simulink model "North_Country_Grid"  (R2025a)
settings: Solver=VariableStepAuto  StartTime=0.0  StopTime=10  RelTol=1e-3
PreLoadFcn:
  | Ts=50e-6;
InitFcn:
  | xInitial = WindFarmType4AverageModelInit;
  | Ts=50e-6;
undefined symbols (not defined in the file): D1, D11, Delta, DiscIntNeverNeededParam, find_system, Fnom_I, Fnom_R, Idc_nom, lagging, level, pulse, test_alpha, Vdc_nom, VLL_nom_I, VLL_nom_R
libraries: spsSecondOrderFilterLib x47, powerlib_extras x38, simulink x34, spsThreePhaseVIMeasurementLib x30, spsFirstOrderFilterLib x29, simulink_extras x26, spsabctodq0Lib x25, spsThreePhaseTransformerTwoWindingsLib x19, spsThreePhaseBreakerLib x18, spsThreePhasePISectionLineLib x17, spsControlledVoltageSourceLib x15, spsOnDelayLib x12
(part 8 of 18)

== system North_Country_Grid/Chateauguay HVDC Back-to-Back Converter/Inverter Control and Protection/Inverter Pole Control (Current//Voltage//Gamma)/Voltage Error ==
  note: Voltage Error
  Vd_ref : Inport
  Vd_meas : Inport  Port=2
  Block : Inport  Port=3
  Id_err : Inport  Port=4
  Enable (Held) : EnablePort  PropagateVarSize=During execution
  Constant1 : Constant  Value=0
  Constant2 : Constant  Value=0
  Constant3 : Constant  Value=Vd_marg
  Constant4 : Constant  Value=Id_marg
  First-Order Filter (T = 0.1) : spsFirstOrderFilterLib/First-Order Filter  FilterType=Lowpass  Tc=0.01  Ts=Ts  Initialize=on  Vac_Init=[0, 0, 60]  Vdc_Init=0  PlotResponse=off  FreqRange="[0,  200,  1]"
  MIN:eps MAX:inf : Saturate  UpperLimit=inf  LowerLimit=eps
  Math Function : Math  Operator=reciprocal  SignedPower=on
  Product1 : Product  Inputs=3  InputSameDT=on  SaturateOnIntegerOverflow=on  OutDataTypeStr=Inherit: Same as first input
  Saturation Dynamic : simulink/Discontinuities/Saturation Dynamic  OutMin=[]  OutMax=[]  OutDataTypeStr=Inherit: Same as second input  OutDataType=fixdt(1, 16)  OutScaling=2^-10  DoSatur=off
  Sum3 : Sum  Inputs=+--  InputSameDT=on  SaturateOnIntegerOverflow=on  OutDataTypeStr=Inherit: Same as first input
  Switch2 : Switch  Criteria=u2 > Threshold
  ERR_V : Outport  VectorParamsAs1DForOutWhenUnconnected=off
  wires:
  Saturation Dynamic/1 -> Product1/3
  Constant3/1 -> Product1/1
  Id_err/1 -> Saturation Dynamic/2
  First-Order Filter (T = 0.1)/1 -> Sum3/3  "dV"
  Product1/1 -> First-Order Filter (T = 0.1)/1
  Constant4/1 -> MIN:eps MAX:inf/1, Saturation Dynamic/1
  MIN:eps MAX:inf/1 -> Math Function/1
  Math Function/1 -> Product1/2
  Constant2/1 -> Saturation Dynamic/3
  Switch2/1 -> ERR_V/1  "ERR"
  Block/1 -> Switch2/2
  Constant1/1 -> Switch2/1
  Vd_meas/1 -> Sum3/2
  Vd_ref/1 -> Sum3/1
  Sum3/1 -> Switch2/3

== system North_Country_Grid/Chateauguay HVDC Back-to-Back Converter/Inverter Control and Protection/Inverter Pole Control (Current//Voltage//Gamma)/Voltage Regulator ==
  note: Voltage Regulator
  Max_i : Inport
  Min_i : Inport  Port=2
  ERR : Inport  Port=3
  Max_pi : Inport  Port=4
  Min_pi : Inport  Port=5
  Alpha_lin : Inport  Port=6
  Max_lin : Inport  Port=7
  Min_lin : Inport  Port=8
  Inv : Inport  Port=9
  Enable (Held) : EnablePort  PropagateVarSize=During execution
  PI Regulator with external limits and linrarized Kp (Discrete) : Subsystem  mask(PI Regulator  With  External  Limits (Discrete)){Kp=Kp_V, Ki=Ki_V, IC_i=ICi_V, On_lin=on, pas=Ts}
      mask prompts: Kp "Kp (deg/pu):"; Ki "Ki (deg/pu/s):"; IC_i "Integrator Initial Condition (deg):"; On_lin "Linearization  (On)"; pas "Sample time (s):"
      mask help: For the linearization it is important to specifie the mode of operation i.e. rectifier or inverter (negation of rectifier).
      mask Display: disp('PI Regulator\nWith external limits\n(Linearized Kp)\n(Discrete)\n\n')
  Alpha_ord : Outport  VectorParamsAs1DForOutWhenUnconnected=off
  wires:
  Inv/1 -> PI Regulator with external limits and linrarized Kp (Discrete)/9(Inv)
  Min_lin/1 -> PI Regulator with external limits and linrarized Kp (Discrete)/8(Min_lin)
  Max_lin/1 -> PI Regulator with external limits and linrarized Kp (Discrete)/7(Max_lin)
  Alpha_lin/1 -> PI Regulator with external limits and linrarized Kp (Discrete)/6(Alpha_lin)
  Min_pi/1 -> PI Regulator with external limits and linrarized Kp (Discrete)/5(Min_pi)
  Max_pi/1 -> PI Regulator with external limits and linrarized Kp (Discrete)/4(Max_pi)
  ERR/1 -> PI Regulator with external limits and linrarized Kp (Discrete)/3(ERR)
  Min_i/1 -> PI Regulator with external limits and linrarized Kp (Discrete)/2(Min_i)
  Max_i/1 -> PI Regulator with external limits and linrarized Kp (Discrete)/1(Max_i)
  PI Regulator with external limits and linrarized Kp (Discrete)/1(Alpha_ord) -> Alpha_ord/1

== system North_Country_Grid/Chateauguay HVDC Back-to-Back Converter/Inverter Control and Protection/Inverter Pole Control (Current//Voltage//Gamma)/Voltage dependent Current Order Limiter ==
  note: Voltage dependent Current Order Limiter (VDCOL) (Discrete)
  Id_ref (pu) : Inport
  Vd (pu) : Inport  Port=2
  Constant : Constant  Value=Id_min
  Constant1 : Constant  Value=Vd_min
  Constant2 : Constant  Value=Vd_seuil
  Constant3 : Constant
  Constant4 : Constant
  Constant5 : Constant  Value=Tu
  Logical Operator : Logic  Operator=NOT
  Low Pass (IC = 1.0) : Subsystem  mask(Low Pass Filter With Reset (discrete: Zoh method, Forward Euler)){ic=1, dt=Ts}
      mask prompts: ic "Initial condition:"; dt "Sample time (s)"
      mask help:
      | The output will be reset to the input value (Time constant = 0)  during the input (2) is True. The Time constant (T) is defined by
      | input (3).
      mask Display:
      | plot(0,0,100,100,[90,80,70,60,50,40,29,20,10],[60,55,52,55,60,65,67,65,60],[89,80,71,60,50,40,30,20,10],[40,35,32,35,40,45,47,45,40],[56,44],[70,50]);
      | disp('\n\nD')
  Math Function : Math  Operator=reciprocal  SignedPower=on
  Max = 10 Min=Id_min_abs : Saturate  UpperLimit=10  LowerLimit=Id_min_abs
  MinMax2 : MinMax  Function=max  Inputs=2  InputSameDT=on  SaturateOnIntegerOverflow=on
  MinMax3 : MinMax  Inputs=2  InputSameDT=on  SaturateOnIntegerOverflow=on
  Product{,1..4} (5 alike) : Product  InputSameDT=on  SaturateOnIntegerOverflow=on  OutDataTypeStr=Inherit: Same as first input
  Relational Operator : RelationalOperator
  Sum : Sum  Inputs=+-  InputSameDT=on  SaturateOnIntegerOverflow=on  OutDataTypeStr=Inherit: Same as first input
  Sum1 : Sum  Inputs=+-  InputSameDT=on  SaturateOnIntegerOverflow=on  OutDataTypeStr=Inherit: Same as first input
  Sum2 : Sum  Inputs=+-  InputSameDT=on  SaturateOnIntegerOverflow=on  OutDataTypeStr=Inherit: Same as first input
  Sum3 : Sum  InputSameDT=on  SaturateOnIntegerOverflow=on  OutDataTypeStr=Inherit: Same as first input
  Unit Delay : UnitDelay  SampleTime=Ts  HasFrameUpgradeWarning=on
  Id_ref_lim : Outport  InitialOutput=0  VectorParamsAs1DForOutWhenUnconnected=off
  Vd_filt : Outport  Port=2  InitialOutput=0  VectorParamsAs1DForOutWhenUnconnected=off
  wires:
  Relational Operator/1 -> Unit Delay/1
  Max = 10 Min=Id_min_abs/1 -> MinMax2/2
  MinMax2/1 -> MinMax3/2
  Product1/1 -> MinMax2/1  "Idref_lim"
  Constant2/1 -> Product3/1, Sum1/1
  Product/1 -> Product3/2, Product2/1  "A"
  Product3/1 -> Sum2/2
  MinMax3/1 -> Id_ref_lim/1
  Id_ref (pu)/1 -> Product4/2, MinMax3/1, Product1/1
  Product4/1 -> Max = 10 Min=Id_min_abs/1  "min"
  Constant/1 -> Product4/1, Sum/2
  Sum3/1 -> Product1/2
  Product2/1 -> Sum3/2
  Sum2/1 -> Sum3/1  "B"
  Constant4/1 -> Sum2/1
  Math Function/1 -> Product/2
  Sum/1 -> Product/1
  Sum1/1 -> Math Function/1
  Constant1/1 -> Sum1/2
  Constant3/1 -> Sum/1
  Constant5/1 -> Low Pass (IC = 1.0)/3(T)
  Low Pass (IC = 1.0)/1(Out) -> Vd_filt/1, Relational Operator/2, Product2/2
  Vd (pu)/1 -> Relational Operator/1, Low Pass (IC = 1.0)/1(In)
  Unit Delay/1 -> Logical Operator/1
  Logical Operator/1 -> Low Pass (IC = 1.0)/2(R)

== system North_Country_Grid/Chateauguay HVDC Back-to-Back Converter/Inverter Control and Protection/Inverter Pole Control (Current//Voltage//Gamma)/alpha_init ==
  In1 : Inport  PortDimensions=1
  IC : InitialCondition  Value=min([ICi_V,ICi_I,ICi_G])
  Out1 : Outport  VectorParamsAs1DForOutWhenUnconnected=off
  wires:
  IC/1 -> Out1/1
  In1/1 -> IC/1

== system North_Country_Grid/Chateauguay HVDC Back-to-Back Converter/Inverter Control and Protection/Inverter Protections/Commutation Failure Prevention Control (CFPREV) ==
  note: Commutation failure Prevention Control Module (CFPREV)
  Uabc (pu) : Inport
  C : Constant  Value=STATE
  CFPREV : Subsystem  TreatAsAtomicUnit=on
  AMIN_CFPREV (deg) : Outport  VectorParamsAs1DForOutWhenUnconnected=off
  wires:
  C/1 -> CFPREV/Enable
  Uabc (pu)/1 -> CFPREV/1(Uabc (pu))
  CFPREV/1(AMIN_CFPREV (deg)) -> AMIN_CFPREV (deg)/1

== system North_Country_Grid/Chateauguay HVDC Back-to-Back Converter/Inverter Control and Protection/Inverter Protections/Informations ==
  note: The CFPREV  mitigates commutation failures due to AC voltage dips. After a fault detection (three-phase or
      | one-phase) an angle value (AMIN_CFPREV) is sent to the converter control in order to be deducted from the
      | maximum delay angle limit (alpha_max). In practice, the commutation margin is consequently enlarged
      | reducing therefore the risk of commutation failures (note 1).
  note: The Commutation failure prevention control (CFPREV) and the Low AC voltage detection (LACVD)
      | constitutes the protective functions at the rinverter.
  note: The LACVD detects a low AC voltage condition on the inverter commutation bus and sends a signal
      | (Lock) to the DCPROT (in the rectifier) in order to prevent the detection of a DC fault when the drop in
      | the DC voltage is due to a fault on the AC side. The LACVD at the irectifier sends also a signal to
      | lock the DCPROT for the same reason.
  note: DESCRIPTION
  note: DC Protections - Inverter
  note: NOTE 1: Result of a failure of the incoming valve to take over the direct current before the commutating voltage reverses its polarity.

== system North_Country_Grid/Chateauguay HVDC Back-to-Back Converter/Inverter Control and Protection/Inverter Protections/Low  AC Voltage Detection (LACVD) ==
  note: Low AC Voltage Detection
  Uac (pu) : Inport
  Enable (Held) : EnablePort  PropagateVarSize=During execution  ShowOutputPort=on
  C : Constant  Value=STATE
  LACVD : Subsystem  TreatAsAtomicUnit=on
  Logical Operator : Logic  AllPortsSameDT=off
  Low_AC_Voltage : Outport  VectorParamsAs1DForOutWhenUnconnected=off
  wires:
  Uac (pu)/1 -> LACVD/1(Uac (pu))
  LACVD/1(Low_AC_Voltage) -> Low_AC_Voltage/1
  Enable (Held)/1 -> Logical Operator/1
  Logical Operator/1 -> LACVD/Enable
  C/1 -> Logical Operator/2

== system North_Country_Grid/Chateauguay HVDC Back-to-Back Converter/Inverter Control and Protection/Inverter Protections/Udio_6p ==
  note: Three-phase full-wave rectification
  Uabc (pu) : Inport
  MinMax : MinMax  Function=max  InputSameDT=on  SaturateOnIntegerOverflow=on
  MinMax1 : MinMax  InputSameDT=on  SaturateOnIntegerOverflow=on
  Sum : Sum  Inputs=+-  InputSameDT=on  SaturateOnIntegerOverflow=on  OutDataTypeStr=Inherit: Same as first input
  conversion pu ac->dc : Gain  Gain=pi/(3*sqrt(3))  SaturateOnIntegerOverflow=on  OutDataTypeStr=Inherit: Same as input  ParamDataTypeStr=Inherit: Same as input
  Udio_6p : Outport  VectorParamsAs1DForOutWhenUnconnected=off
  wires:
  conversion pu ac->dc/1 -> Udio_6p/1
  Sum/1 -> conversion pu ac->dc/1
  Uabc (pu)/1 -> MinMax1/1, MinMax/1
  MinMax/1 -> Sum/1
  MinMax1/1 -> Sum/2

== system North_Country_Grid/Chateauguay HVDC Back-to-Back Converter/Master Control/Start//Stop/S1 ==
  Start : Inport
  Down : Constant  Value=0
  Ramp : FromWorkspace  VariableName="[T_ramp,  U_ramp]"  SampleTime=Ts  ZeroCross=off
  Start-Stop Ramp : RateLimiter  RisingSlewLimit=SS_ramp  FallingSlewLimit=-SS_ramp
  Sum : Sum  InputSameDT=on  SaturateOnIntegerOverflow=on  OutDataTypeStr=Inherit: Same as first input
  Switch : Switch  Criteria=u2 > Threshold  InputSameDT=off
  UP : Constant  Value=Min_ref
  Out1 : Outport  InitialOutput=0  VectorParamsAs1DForOutWhenUnconnected=off
  wires:
  Sum/1 -> Out1/1
  Ramp/1 -> Sum/1
  Start/1 -> Switch/2
  Switch/1 -> Start-Stop Ramp/1
  Down/1 -> Switch/3
  UP/1 -> Switch/1
  Start-Stop Ramp/1 -> Sum/2

== system North_Country_Grid/Chateauguay HVDC Back-to-Back Converter/Rectifier Control and Protection/Rectifier Pole Control (Current)/Alpha Control ==
  note: Alpha Control
  Forced_alpha : Inport
  D_alpha : Inport  Port=2
  Constant1 : Constant  Value=alpha_min
  Constant2 : Constant  Value=alpha_max
  Constant3 : Constant  Value=test_alpha
  Data Type Conversion : DataTypeConversion  OutDataTypeStr=boolean
  Logical Operator : Logic  Operator=OR
  "Rate Limiter (Rate limit) " : RateLimiter  RisingSlewLimit=PRate_fix  FallingSlewLimit=NRate_fix
  "Rate Limiter (Rate limit)    " : RateLimiter  RisingSlewLimit=PRate_fix  FallingSlewLimit=NRate_fix
  Sum : Sum  Inputs=-+  InputSameDT=on  SaturateOnIntegerOverflow=on  OutDataTypeStr=Inherit: Same as first input
  Switch : Switch  Criteria=u2 > Threshold
  Switch1 : Switch  Criteria=u2 > Threshold
  fixed alpha (deg) : Constant  Value=alpha_fix
  Max_i : Outport  VectorParamsAs1DForOutWhenUnconnected=off
  Min_i : Outport  Port=2  VectorParamsAs1DForOutWhenUnconnected=off
  wires:
  "Rate Limiter (Rate limit)    "/1 -> Min_i/1
  "Rate Limiter (Rate limit) "/1 -> Max_i/1
  D_alpha/1 -> Sum/1
  Sum/1 -> Switch/3
  Constant2/1 -> Sum/2
  Constant3/1 -> Logical Operator/1
  Logical Operator/1 -> Switch/2, Switch1/2
  Constant1/1 -> Switch1/3
  Switch/1 -> "Rate Limiter (Rate limit) "/1
  Switch1/1 -> "Rate Limiter (Rate limit)    "/1
  fixed alpha (deg)/1 -> Switch/1, Switch1/1
  Forced_alpha/1 -> Data Type Conversion/1
  Data Type Conversion/1 -> Logical Operator/2

== system North_Country_Grid/Chateauguay HVDC Back-to-Back Converter/Rectifier Control and Protection/Rectifier Pole Control (Current)/Control Mode  ==
  note: AMIN
  note: CONTROL MODE (#):
      |
      | 0) Blocked
      | 1) Current control
      | 2) Voltage control
      | 3) Alpha minimum limitation
      | 4) Alpha maximum limitation
      | 5) Forced or constant Alpha
      | 6) Gamma control
  "a_ord_i " : Inport
  a_ord_v : Inport  Port=2
  a_ord_g : Inport  Port=3
  alpha_ord : Inport  Port=4
  Max_i : Inport  Port=5
  Min_i : Inport  Port=6
  Block : Inport  Port=7
  C : Constant  Value=0
  Data Type Conversion{1..6} (6 alike) : DataTypeConversion  OutDataTypeStr=double  SaturateOnIntegerOverflow=off  RndMeth=Floor
  Gain1 : Gain  Gain=3  OutDataTypeStr=double  SaturateOnIntegerOverflow=on  ParamDataTypeStr=Inherit: Same as input
  Gain2 : Gain  Gain=4  OutDataTypeStr=double  SaturateOnIntegerOverflow=on  ParamDataTypeStr=Inherit: Same as input
  Gain3 : Gain  Gain=2  OutDataTypeStr=double  SaturateOnIntegerOverflow=on  ParamDataTypeStr=Inherit: Same as input
  Gain4 : Gain  Gain=5  OutDataTypeStr=double  SaturateOnIntegerOverflow=on  ParamDataTypeStr=Inherit: Same as input
  Gain5 : Gain  Gain=6  OutDataTypeStr=double  SaturateOnIntegerOverflow=on  ParamDataTypeStr=Inherit: Same as input
  Logical Operator{,1,3,10} (4 alike) : Logic
  Logical Operator2 : Logic  Inputs=3
  Logical Operator4 : Logic  Operator=OR
  Logical Operator{5..7,9} (4 alike) : Logic  Operator=NOT
  Logical Operator8 : Logic  Operator=OR
  MinMax : MinMax  Inputs=2  InputSameDT=on  SaturateOnIntegerOverflow=on
  MinMax1 : MinMax  Inputs=2  InputSameDT=on  SaturateOnIntegerOverflow=on
  Relational Operator : RelationalOperator  Operator=<=
  Relational Operator1 : RelationalOperator  Operator=<=
  Relational Operator2 : RelationalOperator
  Relational Operator3 : RelationalOperator  Operator=<
  Relational Operator4 : RelationalOperator  Operator===
  Sum : Sum  Inputs=++++++  InputSameDT=on  SaturateOnIntegerOverflow=on  OutDataTypeStr=Inherit: Same as first input
  Switch : Switch  Criteria=u2 > Threshold
  mode : Outport  VectorParamsAs1DForOutWhenUnconnected=off
  wires:
  Data Type Conversion6/1 -> Gain4/1
  Data Type Conversion5/1 -> Gain2/1
  Data Type Conversion4/1 -> Gain1/1
  Data Type Conversion3/1 -> Gain5/1
  Data Type Conversion2/1 -> Gain3/1
  Data Type Conversion1/1 -> Sum/1
  Switch/1 -> mode/1
  Logical Operator5/1 -> Logical Operator3/2, Logical Operator/2, Logical Operator10/2
  Logical Operator7/1 -> Logical Operator2/3, Logical Operator1/2
  Gain4/1 -> Sum/5
  Logical Operator1/1 -> Data Type Conversion4/1
  Relational Operator4/1 -> Logical Operator7/1, Data Type Conversion6/1  "AFOR"
  Max_i/1 -> Relational Operator4/2, Relational Operator2/2
  Min_i/1 -> Relational Operator4/1, Relational Operator1/2
  Gain2/1 -> Sum/4
  Gain1/1 -> Sum/3
  Logical Operator2/1 -> Data Type Conversion5/1
  Logical Operator6/1 -> Logical Operator2/1
  Relational Operator2/1 -> Logical Operator2/2, Logical Operator4/2  "AMAX"
  Logical Operator4/1 -> Logical Operator5/1
  Relational Operator1/1 -> Logical Operator1/1, Logical Operator6/1, Logical Operator4/1
  alpha_ord/1 -> Relational Operator2/1, Relational Operator1/1  "alpha_ord"
  Logical Operator/1 -> Data Type Conversion2/1
  Relational Operator3/1 -> Logical Operator/1, Logical Operator8/2  "AVR"
  Gain3/1 -> Sum/2
  Logical Operator3/1 -> Data Type Conversion1/1
  Relational Operator/1 -> Logical Operator3/1, Logical Operator8/1  "ACR"
  "a_ord_i "/1 -> Relational Operator/1, MinMax1/1
  Block/1 -> Switch/2
  Sum/1 -> Switch/3
  C/1 -> Switch/1
  a_ord_v/1 -> MinMax/1, Relational Operator3/1
  a_ord_g/1 -> MinMax/2, MinMax1/2
  MinMax/1 -> Relational Operator/2
  Logical Operator8/1 -> Logical Operator9/1
  Gain5/1 -> Sum/6
  MinMax1/1 -> Relational Operator3/2
  Logical Operator9/1 -> Logical Operator10/1  "AGR"
  Logical Operator10/1 -> Data Type Conversion3/1

== system North_Country_Grid/Chateauguay HVDC Back-to-Back Converter/Rectifier Control and Protection/Rectifier Pole Control (Current)/Current Regulator ==
  note: Current Regulator
  Max_i : Inport
  Min_i : Inport  Port=2
  ERR : Inport  Port=3
  Max_pi : Inport  Port=4
  Min_pi : Inport  Port=5
  Alpha_lin : Inport  Port=6
  Max_lin : Inport  Port=7
  Min_lin : Inport  Port=8
  Inv : Inport  Port=9
  PI Regulator with external limits and linrarized Kp (Discrete) : Subsystem  mask(PI Regulator  With  External  Limits (Discrete)){Kp=Kp_I, Ki=Ki_I, IC_i=ICi_I, On_lin=on, pas=Ts}
      mask prompts: Kp "Kp (deg/pu):"; Ki "Ki (deg/pu/s):"; IC_i "Integrator Initial Condition (deg):"; On_lin "Linearization  (On)"; pas "Sample time (s):"
      mask help: For the linearization it is important to specifie the mode of operation i.e. rectifier or inverter (negation of rectifier).
      mask Display: disp('PI Regulator\nWith external limits\n(Linearized Kp)\n(Discrete)\n\n')
  Alpha_ord : Outport  VectorParamsAs1DForOutWhenUnconnected=off
  wires:
  PI Regulator with external limits and linrarized Kp (Discrete)/1(Alpha_ord) -> Alpha_ord/1
  Max_i/1 -> PI Regulator with external limits and linrarized Kp (Discrete)/1(Max_i)
  Min_i/1 -> PI Regulator with external limits and linrarized Kp (Discrete)/2(Min_i)
  ERR/1 -> PI Regulator with external limits and linrarized Kp (Discrete)/3(ERR)
  Max_pi/1 -> PI Regulator with external limits and linrarized Kp (Discrete)/4(Max_pi)
  Min_pi/1 -> PI Regulator with external limits and linrarized Kp (Discrete)/5(Min_pi)
  Alpha_lin/1 -> PI Regulator with external limits and linrarized Kp (Discrete)/6(Alpha_lin)
  Max_lin/1 -> PI Regulator with external limits and linrarized Kp (Discrete)/7(Max_lin)
  Min_lin/1 -> PI Regulator with external limits and linrarized Kp (Discrete)/8(Min_lin)
  Inv/1 -> PI Regulator with external limits and linrarized Kp (Discrete)/9(Inv)

== system North_Country_Grid/Chateauguay HVDC Back-to-Back Converter/Rectifier Control and Protection/Rectifier Pole Control (Current)/Gamma Error ==
  note: Gamma Error
  G_ref : Inport
  G_meas : Inport  Port=2
  Block : Inport  Port=3
  Id_err : Inport  Port=4
  Enable (Held) : EnablePort  PropagateVarSize=During execution
  Constant1 : Constant  Value=0
  Constant2 : Constant  Value=0
  Constant3 : Constant  Value=G_marg
  Constant4 : Constant  Value=Id_marg
  First-Order Filter (T=0.01) : spsFirstOrderFilterLib/First-Order Filter  FilterType=Lowpass  Tc=0.01  Ts=Ts  Initialize=off  Vac_Init=[0, 0, 60]  Vdc_Init=0  PlotResponse=off  FreqRange="[0,  200,  1]"
  MIN:eps MAX:inf : Saturate  UpperLimit=inf  LowerLimit=eps
  Math Function : Math  Operator=reciprocal  SignedPower=on
  Product1 : Product  Inputs=3  InputSameDT=on  SaturateOnIntegerOverflow=on  OutDataTypeStr=Inherit: Same as first input
  Saturation Dynamic : simulink/Discontinuities/Saturation Dynamic  OutMin=[]  OutMax=[]  OutDataTypeStr=Inherit: Same as second input  OutDataType=fixdt(1, 16)  OutScaling=2^-10  DoSatur=off
  Sum3 : Sum  Inputs=-+-  InputSameDT=on  SaturateOnIntegerOverflow=on  OutDataTypeStr=Inherit: Same as first input
  Switch2 : Switch  Criteria=u2 > Threshold
  ERR_G : Outport  VectorParamsAs1DForOutWhenUnconnected=off
  wires:
  Saturation Dynamic/1 -> Product1/3
  Sum3/1 -> Switch2/3
  G_ref/1 -> Sum3/1
  G_meas/1 -> Sum3/2
  Constant1/1 -> Switch2/1
  Block/1 -> Switch2/2
  Switch2/1 -> ERR_G/1  "ERR"
  Constant2/1 -> Saturation Dynamic/3
  Math Function/1 -> Product1/2
  MIN:eps MAX:inf/1 -> Math Function/1
  Constant4/1 -> MIN:eps MAX:inf/1, Saturation Dynamic/1
  Product1/1 -> First-Order Filter (T=0.01)/1
  First-Order Filter (T=0.01)/1 -> Sum3/3  "dG"
  Id_err/1 -> Saturation Dynamic/2
  Constant3/1 -> Product1/1

== system North_Country_Grid/Chateauguay HVDC Back-to-Back Converter/Rectifier Control and Protection/Rectifier Pole Control (Current)/Gamma Regulator ==
  note: Gamma Regulator
  Max_i : Inport
  Min_i : Inport  Port=2
  ERR : Inport  Port=3
  Max_pi : Inport  Port=4
  Min_pi : Inport  Port=5
  Alpha_lin : Inport  Port=6
  Max_lin : Inport  Port=7
  Min_lin : Inport  Port=8
  Inv : Inport  Port=9
  Enable (Held) : EnablePort  PropagateVarSize=During execution
  PI Regulator with external limits and linrarized Kp (Discrete)1 : Subsystem  mask(PI Regulator  With  External  Limits (Discrete)){Kp=Kp_G, Ki=Ki_G, IC_i=ICi_G, On_lin=on, pas=Ts}
      mask prompts: Kp "Kp (deg/pu):"; Ki "Ki (deg/pu/s):"; IC_i "Integrator Initial Condition (deg):"; On_lin "Linearization  (On)"; pas "Sample time (s):"
      mask help: For the linearization it is important to specifie the mode of operation i.e. rectifier or inverter (negation of rectifier).
      mask Display: disp('PI Regulator\nWith external limits\n(Linearized Kp)\n(Discrete)\n\n')
  Alpha_ord : Outport  VectorParamsAs1DForOutWhenUnconnected=off
  wires:
  PI Regulator with external limits and linrarized Kp (Discrete)1/1(Alpha_ord) -> Alpha_ord/1
  Max_i/1 -> PI Regulator with external limits and linrarized Kp (Discrete)1/1(Max_i)
  Min_i/1 -> PI Regulator with external limits and linrarized Kp (Discrete)1/2(Min_i)
  ERR/1 -> PI Regulator with external limits and linrarized Kp (Discrete)1/3(ERR)
  Max_pi/1 -> PI Regulator with external limits and linrarized Kp (Discrete)1/4(Max_pi)
  Min_pi/1 -> PI Regulator with external limits and linrarized Kp (Discrete)1/5(Min_pi)
  Alpha_lin/1 -> PI Regulator with external limits and linrarized Kp (Discrete)1/6(Alpha_lin)
  Max_lin/1 -> PI Regulator with external limits and linrarized Kp (Discrete)1/7(Max_lin)
  Min_lin/1 -> PI Regulator with external limits and linrarized Kp (Discrete)1/8(Min_lin)
  Inv/1 -> PI Regulator with external limits and linrarized Kp (Discrete)1/9(Inv)

== system North_Country_Grid/Chateauguay HVDC Back-to-Back Converter/Rectifier Control and Protection/Rectifier Pole Control (Current)/Voltage Error ==
  note: Voltage Error
  Vd_ref : Inport
  Vd_meas : Inport  Port=2
  Block : Inport  Port=3
  Id_err : Inport  Port=4
  Enable (Held) : EnablePort  PropagateVarSize=During execution
  Constant1 : Constant  Value=0
  Constant2 : Constant  Value=0
  Constant3 : Constant  Value=Vd_marg
  Constant4 : Constant  Value=Id_marg
  First-Order Filter (T = 0.1) : spsFirstOrderFilterLib/First-Order Filter  FilterType=Lowpass  Tc=0.01  Ts=Ts  Initialize=on  Vac_Init=[0, 0, 60]  Vdc_Init=0  PlotResponse=off  FreqRange="[0,  200,  1]"
  MIN:eps MAX:inf : Saturate  UpperLimit=inf  LowerLimit=eps
  Math Function : Math  Operator=reciprocal  SignedPower=on
  Product1 : Product  Inputs=3  InputSameDT=on  SaturateOnIntegerOverflow=on  OutDataTypeStr=Inherit: Same as first input
  Saturation Dynamic : simulink/Discontinuities/Saturation Dynamic  OutMin=[]  OutMax=[]  OutDataTypeStr=Inherit: Same as second input  OutDataType=fixdt(1, 16)  OutScaling=2^-10  DoSatur=off
  Sum3 : Sum  Inputs=+--  InputSameDT=on  SaturateOnIntegerOverflow=on  OutDataTypeStr=Inherit: Same as first input
  Switch2 : Switch  Criteria=u2 > Threshold
  ERR_V : Outport  VectorParamsAs1DForOutWhenUnconnected=off
  wires:
  Saturation Dynamic/1 -> Product1/3
  Constant3/1 -> Product1/1
  Id_err/1 -> Saturation Dynamic/2
  First-Order Filter (T = 0.1)/1 -> Sum3/3  "dV"
  Product1/1 -> First-Order Filter (T = 0.1)/1
  Constant4/1 -> MIN:eps MAX:inf/1, Saturation Dynamic/1
  MIN:eps MAX:inf/1 -> Math Function/1
  Math Function/1 -> Product1/2
  Constant2/1 -> Saturation Dynamic/3
  Switch2/1 -> ERR_V/1  "ERR"
  Block/1 -> Switch2/2
  Constant1/1 -> Switch2/1
  Vd_meas/1 -> Sum3/2
  Vd_ref/1 -> Sum3/1
  Sum3/1 -> Switch2/3

== system North_Country_Grid/Chateauguay HVDC Back-to-Back Converter/Rectifier Control and Protection/Rectifier Pole Control (Current)/Voltage Regulator ==
  note: Voltage Regulator
  Max_i : Inport
  Min_i : Inport  Port=2
  ERR : Inport  Port=3
  Max_pi : Inport  Port=4
  Min_pi : Inport  Port=5
  Alpha_lin : Inport  Port=6
  Max_lin : Inport  Port=7
  Min_lin : Inport  Port=8
  Inv : Inport  Port=9
  Enable (Held) : EnablePort  PropagateVarSize=During execution
  PI Regulator with external limits and linrarized Kp (Discrete) : Subsystem  mask(PI Regulator  With  External  Limits (Discrete)){Kp=Kp_V, Ki=Ki_V, IC_i=ICi_V, On_lin=on, pas=Ts}
      mask prompts: Kp "Kp (deg/pu):"; Ki "Ki (deg/pu/s):"; IC_i "Integrator Initial Condition (deg):"; On_lin "Linearization  (On)"; pas "Sample time (s):"
      mask help: For the linearization it is important to specifie the mode of operation i.e. rectifier or inverter (negation of rectifier).
      mask Display: disp('PI Regulator\nWith external limits\n(Linearized Kp)\n(Discrete)\n\n')
  Alpha_ord : Outport  VectorParamsAs1DForOutWhenUnconnected=off
  wires:
  Inv/1 -> PI Regulator with external limits and linrarized Kp (Discrete)/9(Inv)
  Min_lin/1 -> PI Regulator with external limits and linrarized Kp (Discrete)/8(Min_lin)
  Max_lin/1 -> PI Regulator with external limits and linrarized Kp (Discrete)/7(Max_lin)
  Alpha_lin/1 -> PI Regulator with external limits and linrarized Kp (Discrete)/6(Alpha_lin)
  Min_pi/1 -> PI Regulator with external limits and linrarized Kp (Discrete)/5(Min_pi)
  Max_pi/1 -> PI Regulator with external limits and linrarized Kp (Discrete)/4(Max_pi)
  ERR/1 -> PI Regulator with external limits and linrarized Kp (Discrete)/3(ERR)
  Min_i/1 -> PI Regulator with external limits and linrarized Kp (Discrete)/2(Min_i)
  Max_i/1 -> PI Regulator with external limits and linrarized Kp (Discrete)/1(Max_i)
  PI Regulator with external limits and linrarized Kp (Discrete)/1(Alpha_ord) -> Alpha_ord/1

== system North_Country_Grid/Chateauguay HVDC Back-to-Back Converter/Rectifier Control and Protection/Rectifier Pole Control (Current)/Voltage dependent Current Order Limiter ==
  note: Voltage dependent Current Order Limiter (VDCOL) (Discrete)
  Id_ref (pu) : Inport
  Vd (pu) : Inport  Port=2
  Constant : Constant  Value=Id_min
  Constant1 : Constant  Value=Vd_min
  Constant2 : Constant  Value=Vd_seuil
  Constant3 : Constant
  Constant4 : Constant
  Constant5 : Constant  Value=Tu
  Logical Operator : Logic  Operator=NOT
  Low Pass (IC = 1.0) : Subsystem  mask(Low Pass Filter With Reset (discrete: Zoh method, Forward Euler)){ic=1, dt=Ts}
      mask prompts: ic "Initial condition:"; dt "Sample time (s)"
      mask help:
      | The output will be reset to the input value (Time constant = 0)  during the input (2) is True. The Time constant (T) is defined by
      | input (3).
      mask Display:
      | plot(0,0,100,100,[90,80,70,60,50,40,29,20,10],[60,55,52,55,60,65,67,65,60],[89,80,71,60,50,40,30,20,10],[40,35,32,35,40,45,47,45,40],[56,44],[70,50]);
      | disp('\n\nD')
  Math Function : Math  Operator=reciprocal  SignedPower=on
  Max = 10 Min=Id_min_abs : Saturate  UpperLimit=10  LowerLimit=Id_min_abs
  MinMax2 : MinMax  Function=max  Inputs=2  InputSameDT=on  SaturateOnIntegerOverflow=on
  MinMax3 : MinMax  Inputs=2  InputSameDT=on  SaturateOnIntegerOverflow=on
  Product{,1..4} (5 alike) : Product  InputSameDT=on  SaturateOnIntegerOverflow=on  OutDataTypeStr=Inherit: Same as first input
  Relational Operator : RelationalOperator
  Sum : Sum  Inputs=+-  InputSameDT=on  SaturateOnIntegerOverflow=on  OutDataTypeStr=Inherit: Same as first input
  Sum1 : Sum  Inputs=+-  InputSameDT=on  SaturateOnIntegerOverflow=on  OutDataTypeStr=Inherit: Same as first input
  Sum2 : Sum  Inputs=+-  InputSameDT=on  SaturateOnIntegerOverflow=on  OutDataTypeStr=Inherit: Same as first input
  Sum3 : Sum  InputSameDT=on  SaturateOnIntegerOverflow=on  OutDataTypeStr=Inherit: Same as first input
  Unit Delay : UnitDelay  SampleTime=Ts  HasFrameUpgradeWarning=on
  Id_ref_lim : Outport  InitialOutput=0  VectorParamsAs1DForOutWhenUnconnected=off
  Vd_filt : Outport  Port=2  InitialOutput=0  VectorParamsAs1DForOutWhenUnconnected=off
  wires:
  Relational Operator/1 -> Unit Delay/1
  Max = 10 Min=Id_min_abs/1 -> MinMax2/2
  MinMax2/1 -> MinMax3/2
  Product1/1 -> MinMax2/1  "Idref_lim"
  Constant2/1 -> Product3/1, Sum1/1
  Product/1 -> Product3/2, Product2/1  "A"
  Product3/1 -> Sum2/2
  MinMax3/1 -> Id_ref_lim/1
  Id_ref (pu)/1 -> Product4/2, MinMax3/1, Product1/1
  Product4/1 -> Max = 10 Min=Id_min_abs/1  "min"
  Constant/1 -> Product4/1, Sum/2
  Sum3/1 -> Product1/2
  Product2/1 -> Sum3/2
  Sum2/1 -> Sum3/1  "B"
  Constant4/1 -> Sum2/1
  Math Function/1 -> Product/2
  Sum/1 -> Product/1
  Sum1/1 -> Math Function/1
  Constant1/1 -> Sum1/2
  Constant3/1 -> Sum/1
  Constant5/1 -> Low Pass (IC = 1.0)/3(T)
  Low Pass (IC = 1.0)/1(Out) -> Vd_filt/1, Relational Operator/2, Product2/2
  Vd (pu)/1 -> Relational Operator/1, Low Pass (IC = 1.0)/1(In)
  Unit Delay/1 -> Logical Operator/1
  Logical Operator/1 -> Low Pass (IC = 1.0)/2(R)

== system North_Country_Grid/Chateauguay HVDC Back-to-Back Converter/Rectifier Control and Protection/Rectifier Pole Control (Current)/alpha_init ==
  In1 : Inport  PortDimensions=1
  IC : InitialCondition  Value=min([ICi_V,ICi_I,ICi_G])
  Out1 : Outport  VectorParamsAs1DForOutWhenUnconnected=off
  wires:
  IC/1 -> Out1/1
  In1/1 -> IC/1

== system North_Country_Grid/Chateauguay HVDC Back-to-Back Converter/Rectifier Control and Protection/Rectifier Protections/DC Fault Protection (DCPROT) ==
  note: DC Fault Protection (only in Rectifier)
  VdL (pu) : Inport
  Deblocked : Inport  Port=2  OutDataTypeStr=boolean
  Lock : Inport  Port=3
  (Held) : EnablePort  PropagateVarSize=During execution  ShowOutputPort=on
  C : Constant  Value=STATE
  Enabled Subsystem : Subsystem  TreatAsAtomicUnit=on
  Logical Operator : Logic  AllPortsSameDT=off
  Forced_alpha : Outport  VectorParamsAs1DForOutWhenUnconnected=off
  wires:
  (Held)/1 -> Logical Operator/1
  C/1 -> Logical Operator/2
  Logical Operator/1 -> Enabled Subsystem/Enable
  VdL (pu)/1 -> Enabled Subsystem/1(VdL (pu))
  Lock/1 -> Enabled Subsystem/3(Lock)
  Deblocked/1 -> Enabled Subsystem/2(Deblocked)
  Enabled Subsystem/1(Forced_alpha) -> Forced_alpha/1

== system North_Country_Grid/Chateauguay HVDC Back-to-Back Converter/Rectifier Control and Protection/Rectifier Protections/Informations ==
  note: The  DCPROT detects a fault on the DC line and tries to extinguish the fault current by ordering a Forced
      | alpha operation for a fixed duration.
  note: The LACVD detects a low AC voltage condition on the rectifier commutation bus and sends a signal
      | (Lock) to the DCPROT in order to prevent the detection of a DC fault when the drop in the DC voltage is
      | due to a fault on the AC side. The LACVD at the inverter sends also a signal to lock the DCPROT for the
      | same reason.
  note: DC Protections - Rectifier
  note: Silvano Casoria (Hydro-Quebec)
  note: DESCRIPTION
  note: The DC fault protection (DCPROT) and the Low AC voltage detection (LACVD) constitutes the
      | protectives functions at the rectifier. The DC fault protection detects a fault on the DC line and tries to
      | extinguish the fault current by ordering a Forced alpha operation during a fixed duration.

== system North_Country_Grid/Chateauguay HVDC Back-to-Back Converter/Rectifier Control and Protection/Rectifier Protections/Low  AC Voltage Detection (LACVD) ==
  note: Low AC Voltage Detection
  Uac (pu) : Inport
  Enable (Held) : EnablePort  PropagateVarSize=During execution  ShowOutputPort=on
  C : Constant  Value=STATE
  LACVD : Subsystem  TreatAsAtomicUnit=on
  Logical Operator : Logic  AllPortsSameDT=off
  Low_AC_Voltage : Outport  VectorParamsAs1DForOutWhenUnconnected=off
  wires:
  Uac (pu)/1 -> LACVD/1(Uac (pu))
  LACVD/1(Low_AC_Voltage) -> Low_AC_Voltage/1
  Enable (Held)/1 -> Logical Operator/1
  Logical Operator/1 -> LACVD/Enable
  C/1 -> Logical Operator/2

== system North_Country_Grid/Chateauguay HVDC Back-to-Back Converter/Rectifier Control and Protection/Rectifier Protections/Udio_6p ==
  note: Three-phase full-wave rectification
  Uabc (pu) : Inport
  MinMax : MinMax  Function=max  InputSameDT=on  SaturateOnIntegerOverflow=on
  MinMax1 : MinMax  InputSameDT=on  SaturateOnIntegerOverflow=on
  Sum : Sum  Inputs=+-  InputSameDT=on  SaturateOnIntegerOverflow=on  OutDataTypeStr=Inherit: Same as first input
  conversion pu ac->dc : Gain  Gain=pi/(3*sqrt(3))  SaturateOnIntegerOverflow=on  OutDataTypeStr=Inherit: Same as input  ParamDataTypeStr=Inherit: Same as input
  Udio_6p : Outport  VectorParamsAs1DForOutWhenUnconnected=off
  wires:
  conversion pu ac->dc/1 -> Udio_6p/1
  Sum/1 -> conversion pu ac->dc/1
  Uabc (pu)/1 -> MinMax1/1, MinMax/1
  MinMax/1 -> Sum/1
  MinMax1/1 -> Sum/2

== system North_Country_Grid/Jericho Rise (Type 3, 77.7 MW)/DFIG Wind Turbine/Control/Grid-side Controls ==
  note: Uctrl grid converter
  note: Modulation index & phase
  note: Current regulator
  note: Vdc regulator
  note: Required value for modulation index "m" to obtain 1 pu generated voltage by the converter:
  note: m = Vnom * 2*sqrt(2/3) / Vdc
  note: Where Vnom = RMS ph-ph nominal voltage
  note: Wind Turbine controls - Grid-side converter control system
  Iq_ref : Inport
  Idq_gc : Inport  Port=2
  w : Inport  Port=3
  Vdqs : Inport  Port=4
  Vdc : Inport  Port=5
  Theta_PLL : Inport  Port=6
  ->pu : Gain  Gain=1/Vdc_nom
  0-Mod_index_max_grid : Saturate  UpperLimit=Mod_index_max_grid  LowerLimit=0
  Avoid division by zero : Saturate  UpperLimit=inf  LowerLimit=1e-6
  Cartesian to Polar1 : simulink_extras/Transformations/Cartesian to Polar
  Constant1 : Constant  Value=L_RL
  Constant2 : Constant  Value=L_RL
  Constant3 : Constant  Value=R_RL
  Constant4 : Constant  Value=R_RL
  Demux{,1..3} (4 alike) : Demux  Outputs=2
      settings: DisplayOption=none
  Discrete PI Controller : powerlib_extras/Discrete  Control Blocks/Discrete PI Controller  Kp=Kp_dc  Ki=Ki_dc  Par_Limits=[1 -1]*Imax_grid_conv  Init=0  Ts=Ts
  Discrete PI Controller1 : powerlib_extras/Discrete  Control Blocks/Discrete PI Controller  Kp=Kp_grid_side_cur_reg  Ki=Ki_grid_side_cur_reg  Par_Limits=[1.0 -1.0] *Lim_grid_side_cur_reg  Init=0  Ts=Ts
  K : Constant  Value=Vnom*2*sqrt(2/3)
  Mux : Mux  Inputs=2
  Mux2 : Mux  Inputs=2
  Mux4 : Mux  Inputs=3
  Mux5 : Mux  Inputs=2
  Polar to Cartesian : simulink_extras/Transformations/Polar to Cartesian
  Product : Product  Inputs=3  InputSameDT=on  SaturateOnIntegerOverflow=on  OutDataTypeStr=Inherit: Same as first input
  Product1 : Product  Inputs=3  InputSameDT=on  SaturateOnIntegerOverflow=on  OutDataTypeStr=Inherit: Same as first input
  Product2 : Product  InputSameDT=on  SaturateOnIntegerOverflow=on  OutDataTypeStr=Inherit: Same as first input
  Product3 : Product  InputSameDT=on  SaturateOnIntegerOverflow=on  OutDataTypeStr=Inherit: Same as first input
  Product4 : Product  Inputs=**/  InputSameDT=on  SaturateOnIntegerOverflow=on  OutDataTypeStr=Inherit: Same as first input
  Sum1 : Sum  Inputs=+-  InputSameDT=on  SaturateOnIntegerOverflow=on  OutDataTypeStr=Inherit: Same as first input
  Sum2 : Sum  Inputs=-+|  InputSameDT=on  SaturateOnIntegerOverflow=on  OutDataTypeStr=Inherit: Same as first input
  Sum3 : Sum  Inputs=||++-  InputSameDT=on  SaturateOnIntegerOverflow=on  OutDataTypeStr=Inherit: Same as first input
  Sum4 : Sum  Inputs=|+-  InputSameDT=on  SaturateOnIntegerOverflow=on  OutDataTypeStr=Inherit: Same as first input
  Sum5 : Sum  Inputs=|--+  InputSameDT=on  SaturateOnIntegerOverflow=on  OutDataTypeStr=Inherit: Same as first input
  Sum6 : Sum  Inputs=|-+  InputSameDT=on  SaturateOnIntegerOverflow=on  OutDataTypeStr=Inherit: Same as first input
  Sum7 : Sum  Inputs=|+-  InputSameDT=on  SaturateOnIntegerOverflow=on  OutDataTypeStr=Inherit: Same as first input
  Trigonometric Function2 : Trigonometry
  Trigonometric Function3 : Trigonometry  Operator=cos
  V0 : Constant  Value=0
  Vdc_ref (V) : Constant  Value=Vdc_nom
  dq0_to_abc Transformation : powerlib_extras/Measurements/dq0_to_abc Transformation
  Uctrl_grid_conv : Outport  VectorParamsAs1DForOutWhenUnconnected=off
  wires:
  Sum6/1 -> Cartesian to Polar1/2  "Vq_ctrl_grid_conv"
  Sum1/1 -> Cartesian to Polar1/1  "Vd_ctrl_grid_conv"
  dq0_to_abc Transformation/1 -> Uctrl_grid_conv/1
  Theta_PLL/1 -> Trigonometric Function2/1, Trigonometric Function3/1
  Mux4/1 -> dq0_to_abc Transformation/1  "Vdq0"
  Polar to Cartesian/2 -> Mux4/2
  Polar to Cartesian/1 -> Mux4/1
  V0/1 -> Mux4/3
  Trigonometric Function3/1 -> Mux5/2
  Trigonometric Function2/1 -> Mux5/1
  Mux5/1 -> dq0_to_abc Transformation/2
  [Vdc] -> Avoid division by zero/1
  Product4/1 -> 0-Mod_index_max_grid/1  "m"
  K/1 -> Product4/2
  Avoid division by zero/1 -> Product4/3
  Cartesian to Polar1/1 -> Product4/1
  0-Mod_index_max_grid/1 -> Polar to Cartesian/1
  Cartesian to Polar1/2 -> Polar to Cartesian/2
  Mux/1 -> Demux1/1
  Idq_gc/1 -> Demux/1
  w/1 -> [w]
  Constant2/1 -> Product1/2
  Discrete PI Controller1/1 -> Demux3/1
  Mux2/1 -> Discrete PI Controller1/1
  Demux2/1 -> Sum3/1  "Vd"
  Constant1/1 -> Product/1
  Vdqs/1 -> Demux2/1
  Demux/2 -> Sum2/1  "Iq"
  Demux/1 -> Sum4/2  "Id"
  Product/1 -> Sum3/2
  Constant3/1 -> Product2/1
  Constant4/1 -> Product3/2
  Product1/1 -> Sum5/2
  Demux2/2 -> Sum5/3  "Vq"
  Product2/1 -> Sum3/3
  Product3/1 -> Sum5/1
  Sum4/1 -> Mux2/1
  Sum2/1 -> Mux2/2
  [w] -> Product1/3
  [w] -> Product/2
  [iq_ref] -> Product/3
  [id_ref] -> Product2/2
  [iq_ref] -> Product3/1
  [id_ref] -> Product1/1
  Demux3/1 -> Sum1/2  "vd'"
  Demux3/2 -> Sum6/1  "vq'"
  Demux1/2 -> [iq_ref], Sum2/2  "Iq_ref"
  Demux1/1 -> Sum4/1, [id_ref]  "Id_ref"
  Sum3/1 -> Sum1/1
  Sum5/1 -> Sum6/2
  Discrete PI Controller/1 -> Mux/1  "Id_ref"
  Sum7/1 -> ->pu/1
  ->pu/1 -> Discrete PI Controller/1
  Vdc/1 -> [Vdc], Sum7/2
  Iq_ref/1 -> Mux/2  "Iq_ref"
  Vdc_ref (V)/1 -> Sum7/1

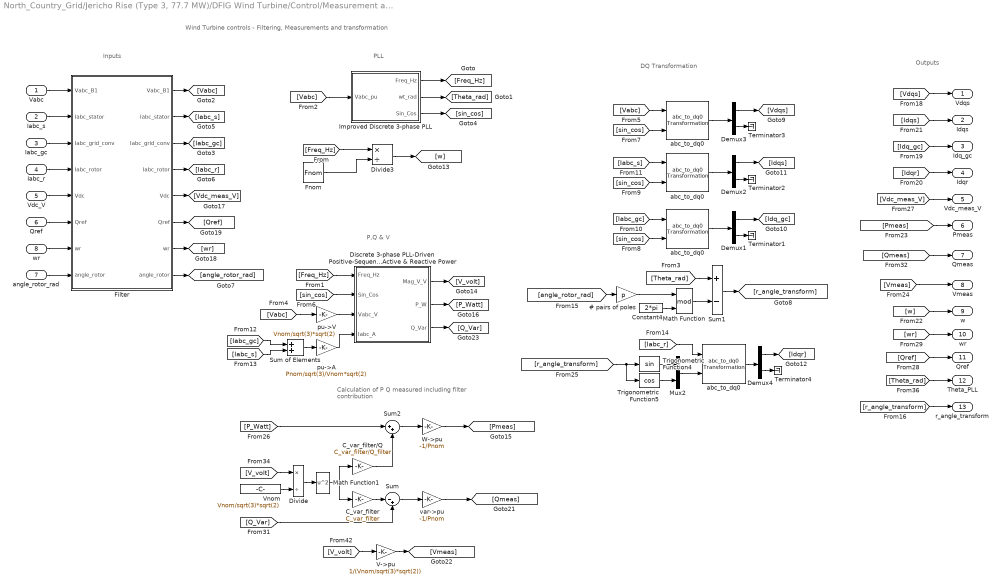
== system North_Country_Grid/Jericho Rise (Type 3, 77.7 MW)/DFIG Wind Turbine/Control/Measurement and Transformation ==
  note: DQ Transformation
  note: P,Q & V
  note: PLL
  note: Inputs
  note: Outputs
  note: Calculation of P Q measured
      | including filter contribution
  note: Wind Turbine controls - Filtering, Measurements and transformation
  Vabc : Inport
  Iabc_s : Inport  Port=2
  Iabc_gc : Inport  Port=3
  Iabc_r : Inport  Port=4
  Vdc_V : Inport  Port=5
  Qref : Inport  Port=6
  angle_rotor_rad : Inport  Port=7
  wr : Inport  Port=8
  "   abc_to_dq0    " : powerlib_extras/Measurements/abc_to_dq0 Transformation
  " Improved Discrete 3-phase PLL" : Subsystem  mask(Discrete 3-phase PLL){Fmin=0.75*Fnom, Par_Init=[0 Fnom], ParK=[5 3.2 1 50], Ts=Ts}
      mask prompts: Fmin "Minimum frequency (Hz):"; Par_Init "Initial inputs:[ Phase(degrees)   Frequency(Hz) ]"; ParK "Regulator gains [ Kp1 Kp2  Ki1  Ki2 ]"; Ts "Sample time:"
      mask help:
      | This Phase Locked Loop (PLL) system can be used  to synchronize on a set of variable frequency, three-phase sinusoidal signals.
      |
      | Input 1: Vector containing the normalized
      |              three-phase signals [Va Vb Vc]
      | Output 1:  Measured frequency (Hz) = w/(2pi)
      | Output 2:  Ramp w.t   varying between  0 and 2*pi,
      | synchronized on zero crossings of the fundamental (positive-sequence) of phase A.
      | Output 3: Vector [sin(wt) cos(wt)]
      mask init:
      | Kp1=ParK(1);
      | Kp2=ParK(2);
      | Ki1=ParK(3);
      | Ki2=ParK(4);
      | Phase_Init=Par_Init(1);
      | Finit=Par_Init(2);
      | power_initmask();
      settings: OpenFcn=power_openblockproxy();
  # pairs of poles : Gain  Gain=p  SaturateOnIntegerOverflow=on  OutDataTypeStr=Inherit: Same as input  ParamDataTypeStr=Inherit: Same as input
  C_var_filter : Gain  Gain=C_var_filter  SaturateOnIntegerOverflow=on  OutDataTypeStr=Inherit: Same as input  ParamDataTypeStr=Inherit: Same as input
  C_var_filter/Q : Gain  Gain=C_var_filter/Q_filter  SaturateOnIntegerOverflow=on  OutDataTypeStr=Inherit: Same as input  ParamDataTypeStr=Inherit: Same as input
  Constant4 : Constant  Value=2*pi
  Demux{1..4} (4 alike) : Demux  Outputs=[2 1]
      settings: DisplayOption=none
  Discrete 3-phase PLL-Driven Positive-Sequence Active & Reactive Power : Subsystem  mask(Discrete 3-phase PLL-Driven Positive-Sequence Active & Reactive Power){Finit=Fnom, Fmin=Fnom*45/60, Par_Vinit=[Vnom/sqrt(3)*sqrt(2) 30], Par_Iinit=[Pnom/sqrt(3)/Vnom*sqrt(2) -10], Ts=Ts}
      mask prompts: Finit "Initial frequency (Hz):"; Fmin "Minimum frequency (Hz):"; Par_Vinit "Voltage initial input: [ Mag  Phase(Degrees) ]"; Par_Iinit "Current initial input: [ Mag  Phase(Degrees) ]"; Ts "Sample time:"
      mask help:
      | This discrete block measures the 3-phase active power P and reactive power Q  associated with a periodic set of 3-phase voltages and currents which may contain harmonics. P and Q are calculated by evaluating the fundamental values (positive-sequence) of the input voltages and currents with a running window over one cycle of the specified frequency (port Freq).
      |  Input port "Sin_Cos" (a two-dimension signal) provides the reference frame required for the computation.
      |
      | input 1: must give the frequency of the fundamental (Hz)
      | Input 2: must contain a  [sin(wt)  cos(wt)] two dimension signal , where w is the rotation speed (rad/s) of the reference frame used for the computation..
      | input 3: Vectorized 3-phase  instantaneous voltage (Vabc)
      | input 4: Vectorized 3-phase instantaneous current (Iabc)
      |
      | Output 1: Vector [Mag_V Mag_I] of the fundamental values (Magnitude) of the voltage & current (peak values of the positive-sequence)
      | Output 2: 3-phase PQ measurement vector [P(W) Q (var)] evaluated at the specified frequency. Current flowing into an RL circuit will produce  positive active and reactive powers.
      |
      | For the first cycle of simulation, the outputs are held constant using the values specified by the parameters "Initial input".
      | he value of the parameter "Minimum frequency" is used to determine the buffer size of the "Variable Transport Delay" block found inside this subsystem.
      mask init:
      | power_initmask();
      settings: OpenFcn=power_openblockproxy();
  Divide : Product  Inputs=*/
  Divide3 : Product  Inputs=*/
  Filter : Subsystem  mask{Freq=Freq_filter, Zeta1=Zeta_filter, Ts=Ts}
      mask prompts: Freq "Cut-off frequency (Hz):"; Zeta1 "Damping factor Zeta:"; Ts "Sample time"
  Fnom : Constant  Value=Fnom
  Math Function : Math  Operator=mod  SignedPower=on
  Math Function1 : Math  Operator=square  SignedPower=on
  Mux2 : Mux  Inputs=2
  Sum : Sum  Inputs=|-+
  Sum of Elements : Sum
  Sum1 : Sum  Inputs=+-  InputSameDT=on  SaturateOnIntegerOverflow=on  OutDataTypeStr=Inherit: Same as first input
  Sum2 : Sum  Inputs=|++
  Terminator{1..4} (4 alike) : Terminator
  Trigonometric Function4 : Trigonometry
  Trigonometric Function5 : Trigonometry  Operator=cos
  V->pu : Gain  Gain=1/(Vnom/sqrt(3)*sqrt(2))  SaturateOnIntegerOverflow=on  OutDataTypeStr=Inherit: Same as input  ParamDataTypeStr=Inherit: Same as input
  Vnom : Constant  Value=Vnom/sqrt(3)*sqrt(2)
  W->pu : Gain  Gain=-1/Pnom  SaturateOnIntegerOverflow=on  OutDataTypeStr=Inherit: Same as input  ParamDataTypeStr=Inherit: Same as input
  abc_to_dq0 : powerlib_extras/Measurements/abc_to_dq0 Transformation
  "abc_to_dq0 " : powerlib_extras/Measurements/abc_to_dq0 Transformation
  "abc_to_dq0  " : powerlib_extras/Measurements/abc_to_dq0 Transformation
  pu->A : Gain  Gain=Pnom/sqrt(3)/Vnom*sqrt(2)  SaturateOnIntegerOverflow=on  OutDataTypeStr=Inherit: Same as input  ParamDataTypeStr=Inherit: Same as input
  pu->V : Gain  Gain=Vnom/sqrt(3)*sqrt(2)  SaturateOnIntegerOverflow=on  OutDataTypeStr=Inherit: Same as input  ParamDataTypeStr=Inherit: Same as input
  "var->pu " : Gain  Gain=-1/Pnom  SaturateOnIntegerOverflow=on  OutDataTypeStr=Inherit: Same as input  ParamDataTypeStr=Inherit: Same as input
  Vdqs : Outport  VectorParamsAs1DForOutWhenUnconnected=off
  Idqs : Outport  Port=2  VectorParamsAs1DForOutWhenUnconnected=off
  Idq_gc : Outport  Port=3  VectorParamsAs1DForOutWhenUnconnected=off
  Idqr : Outport  Port=4  VectorParamsAs1DForOutWhenUnconnected=off
  Vdc_meas_V : Outport  Port=5  VectorParamsAs1DForOutWhenUnconnected=off
  Pmeas : Outport  Port=6  VectorParamsAs1DForOutWhenUnconnected=off
  Qmeas : Outport  Port=7  VectorParamsAs1DForOutWhenUnconnected=off
  Vmeas : Outport  Port=8  VectorParamsAs1DForOutWhenUnconnected=off
  w : Outport  Port=9  VectorParamsAs1DForOutWhenUnconnected=off
  "wr " : Outport  Port=10  VectorParamsAs1DForOutWhenUnconnected=off
  "Qref " : Outport  Port=11  VectorParamsAs1DForOutWhenUnconnected=off
  Theta_PLL : Outport  Port=12  VectorParamsAs1DForOutWhenUnconnected=off
  r_angle_transform : Outport  Port=13  VectorParamsAs1DForOutWhenUnconnected=off
  wires:
  " Improved Discrete 3-phase PLL"/3(Sin_Cos) -> [sin_cos]
  " Improved Discrete 3-phase PLL"/2(wt_rad) -> [Theta_rad]
  " Improved Discrete 3-phase PLL"/1(Freq_Hz) -> [Freq_Hz]
  [Vabc] -> " Improved Discrete 3-phase PLL"/1(Vabc_pu)
  [r_angle_transform] -> r_angle_transform/1
  [V_volt] -> V->pu/1
  V->pu/1 -> [Vmeas]
  [Theta_rad] -> Theta_PLL/1
  [Qmeas] -> Qmeas/1
  Discrete 3-phase PLL-Driven Positive-Sequence Active & Reactive Power/2(P_W) -> [P_Watt]
  Discrete 3-phase PLL-Driven Positive-Sequence Active & Reactive Power/1(Mag_V_V) -> [V_volt]
  Demux1/2 -> Terminator1/1
  Demux3/1 -> [Vdqs]
  Demux3/2 -> Terminator3/1
  "abc_to_dq0  "/1 -> Demux1/1
  abc_to_dq0/1 -> Demux3/1
  Math Function/1 -> Sum1/2
  # pairs of poles/1 -> Math Function/1
  Constant4/1 -> Math Function/2
  Demux4/1 -> [Idqr]
  Demux4/2 -> Terminator4/1
  "   abc_to_dq0    "/1 -> Demux4/1
  Demux2/2 -> Terminator2/1
  Trigonometric Function5/1 -> Mux2/2
  Trigonometric Function4/1 -> Mux2/1
  "abc_to_dq0 "/1 -> Demux2/1
  Fnom/1 -> Divide3/2
  Divide3/1 -> [w]
  Sum of Elements/1 -> pu->A/1
  pu->V/1 -> Discrete 3-phase PLL-Driven Positive-Sequence Active & Reactive Power/3(Vabc_V)
  [Freq_Hz] -> Divide3/1
  [Freq_Hz] -> Discrete 3-phase PLL-Driven Positive-Sequence Active & Reactive Power/1(Freq_Hz)
  [Vabc] -> pu->V/1
  [Vabc] -> abc_to_dq0/1
  [sin_cos] -> Discrete 3-phase PLL-Driven Positive-Sequence Active & Reactive Power/2(Sin_Cos)
  [sin_cos] -> abc_to_dq0/2
  [sin_cos] -> "abc_to_dq0  "/2
  [sin_cos] -> "abc_to_dq0 "/2
  [angle_rotor_rad] -> # pairs of poles/1
  [Iabc_gc] -> "abc_to_dq0  "/1
  [Iabc_s] -> "abc_to_dq0 "/1
  [Iabc_s] -> Sum of Elements/2
  [Iabc_r] -> "   abc_to_dq0    "/1
  Demux1/1 -> [Idq_gc]
  Demux2/1 -> [Idqs]
  [Vdqs] -> Vdqs/1
  [Idq_gc] -> Idq_gc/1
  [Idqr] -> Idqr/1
  [Idqs] -> Idqs/1
  [w] -> w/1
  [Pmeas] -> Pmeas/1
  [Vmeas] -> Vmeas/1
  pu->A/1 -> Discrete 3-phase PLL-Driven Positive-Sequence Active & Reactive Power/4(Iabc_A)
  Sum1/1 -> [r_angle_transform]
  Mux2/1 -> "   abc_to_dq0    "/2
  [r_angle_transform] -> Trigonometric Function4/1, Trigonometric Function5/1
  Vabc/1 -> Filter/1(Vabc_B1)
  Iabc_s/1 -> Filter/2(Iabc_stator)
  Iabc_gc/1 -> Filter/3(Iabc_grid_conv)
  Iabc_r/1 -> Filter/4(Iabc_rotor)
  Vdc_V/1 -> Filter/5(Vdc)
  Qref/1 -> Filter/6(Qref)
  wr/1 -> Filter/7(wr)
  [Vdc_meas_V] -> Vdc_meas_V/1
  [Qref] -> "Qref "/1
  [wr] -> "wr "/1
  "var->pu "/1 -> [Qmeas]
  [Q_Var] -> Sum/2
  W->pu/1 -> [Pmeas]
  [P_Watt] -> Sum2/1
  [V_volt] -> Divide/1
  Vnom/1 -> Divide/2
  Divide/1 -> Math Function1/1
  C_var_filter/1 -> Sum/1
  Sum/1 -> "var->pu "/1
  C_var_filter/Q/1 -> Sum2/2
  Sum2/1 -> W->pu/1
  Math Function1/1 -> C_var_filter/Q/1, C_var_filter/1
  Filter/1("Vabc_B1 ") -> [Vabc]
  Filter/2("Iabc_stator ") -> [Iabc_s]
  Filter/3("Iabc_grid_conv ") -> [Iabc_gc]
  Filter/4("Iabc_rotor ") -> [Iabc_r]
  Filter/5("Vdc ") -> [Vdc_meas_V]
  Filter/6("Qref ") -> [Qref]
  Filter/7("wr ") -> [wr]
  Filter/8("angle_rotor ") -> [angle_rotor_rad]
  angle_rotor_rad/1 -> Filter/8(angle_rotor)
  [Iabc_gc] -> Sum of Elements/1
  Discrete 3-phase PLL-Driven Positive-Sequence Active & Reactive Power/3(Q_Var) -> [Q_Var]
  [Theta_rad] -> Sum1/1
